simulink model "Model_14Bus_AC_DC_Microgrid"  (R2025a)
settings: Solver=ode23tb  StartTime=0.0  StopTime=0.1  MaxStep=1e-2  RelTol=1e-3
InitFcn:
  | Set_parameters_R2018
StopFcn:
  | Save_Data;
  | Graphics;
undefined symbols (not defined in the file): Clink, D1, Delta, dis1, dis10, dis11, dis12, dis13, dis14, dis2, dis3, dis4, dis5, dis6, dis7, dis8, dis9, Fc, Fnom, Hydride, Increment_MPPT, Ion, Ki_Ireg, Ki_VDCreg, Kp_Ireg, Kp_VDCreg, LimitL_Ireg, LimitL_VDCreg, Limits_MPPT, LimitU_Ireg, LimitU_VDCreg, Lithium, max_min, Metal, Nickel, P_Load_2, P_Load_3, Pnom, Pnom_T1, Pnom_T2, Pnom_T3, Pnom_xfo, Ql_Load_2, Ql_Load_3, R_Load_9, R_Load_DC, RL, Rl, RLff, Rls, sigbuilder_block, Ts, Ts_Control, Ts_Power, V1_LL_T3, Vf, Vfd, Vnom_dc, Vnom_DC, Vnom_Diesel ... (+5)
libraries: spsRMSLib x87, spsCurrentMeasurementLib x47, spsThreePhaseVIMeasurementLib x23, spsVoltageMeasurementLib x21, spsPowerLib x21, spsTHDLib x20, spsThreePhaseSeriesRLCBranchLib x20, spsSeriesRLCBranchLib x19, spsIGBTDiodeLib x14, spsThreePhaseBreakerLib x14, powerlib_extras x14, simulink x12
(part 4 of 9)

== system Model_14Bus_AC_DC_Microgrid/Bus_slack  ==
  note: C
  note: B
  note: A
  note: C
  note: Linea - Neutro
  note: B
  note: A
  note: A
  note: B
  note: C
  Conv pu1 : Gain  Gain=sqrt (3) /Vnom_prim  SaturateOnIntegerOverflow=on  OutDataTypeStr=Inherit: Same as input  ParamDataTypeStr=Inherit: Same as input
  Conv pu2 : Gain  Gain=sqrt (3) /Vnom_prim  SaturateOnIntegerOverflow=on  OutDataTypeStr=Inherit: Same as input  ParamDataTypeStr=Inherit: Same as input
  Measurement1 : Scope  NumInputPorts=4
      settings: SampleTime=Ts  Title=Active Powers (W)  ActiveDisplayYMinimum=-103868.59895  ActiveDisplayYMaximum=934817.39056  DataLoggingVariableName=ScopeData39  DataLoggingSaveFormat=Array
  PLL : Subsystem
  PLL (3ph) : spsPLL3phLib/PLL (3ph)  Fmin=45  Par_Init=[0, 60]  ParK=[180, 3200, 1]  TcD=1e-4  MaxRateChangeFreq=12  FilterCutOffFreq=25  Ts=0  AGC=on
  Power Factor Block1 : Subsystem  mask(Power Factor Block){Freq=Fnom, Vinit=[0, 0], Iinit=[0, 0], Ts=0}
      mask prompts: Freq "Fundamental frequency (Hz):"; Vinit "Voltage initial input [ Mag, Phase (degrees) ]:"; Iinit "Current initial input [ Mag, Phase (degrees) ]:"; Ts "Sample time:"
      mask help:
      | Power Factor Block developed by Dr Rodney Tan
      | Version 1.01 (Aug 2016)
      |
      | Compute power factor and phase angle of AC circuit voltage-current pair at fundamental frequency.
      |
      | The computation is based on Power block and Complex number function block.
      |
      | For the first cycle of simulation, the outputs are held constant to the powers computed for the Voltage initial input and Current initial input parameters.
      mask Help:
      | <b>Fundamental Frequency (Hz)</b>
      | Specify the measurement fundamental frequency, in hertz, of the input signal.
      | 
      | <b>Voltage initial input [ Mag, Phase (degrees) ]</b>
      | Specify the voltage initial magnitude and phase to set a constant output for the first cycle of simulation.
      | 
      | <b>Current initial input [ Mag, Phase (degrees) ]</b>
      | Specify the current initial magnitude and phase to set a constant output for the first cycle of simulation.
      | 
      | <b>Sample Time</b>
      | Specify the sample time of the block, in seconds. Set to 0 to implement a continuous block.
      mask TypeOptions Freq: Power/Freq
      mask TypeOptions Vinit: Power/Vinit
      mask TypeOptions Iinit: Power/Iinit
      mask TypeOptions Ts: Power/Ts
  Power Factor1 : Display
  Scope : Scope
      settings: ActiveDisplayYMinimum=-56.88569  ActiveDisplayYMaximum=237.8062
  Scope2 : Scope
      settings: DataLoggingVariableName=ScopeData3
  THD : spsTHDLib/THD  Freq=60  Ts=Ts_Power
  THD (% and signal) : Scope  NumInputPorts=2
      settings: TimeSpan=0.1  ActiveDisplayYMinimum=-21318.64578  ActiveDisplayYMaximum=21318.87173
  THD (%) : Display
      settings: Format=bank
  Terminator : Terminator
  Vabc pu1 : Scope
      settings: TimeSpan=3  Title=Vabc_Instantaneo y rms (pu)  ActiveDisplayYMinimum=-1.96658  ActiveDisplayYMaximum=2.46633  DataLoggingVariableName=ScopeData40
  frecuency (Hz) : Display
  to % : Gain  Gain=100  SampleTime=Ts_Power
  ángulo de V (%)1 : Display
      settings: Format=bank
  tag scope: PFabc_Bus13=global, THDv_abc_Bus13=global, delta_abc_Bus13=global
  wires:
  [Iabc_Sec] -> Power Factor Block1/2(Iabc)  "Signal Iabc"
  THD/1 -> to %/1
  Power Factor Block1/4(Iabc y Iabc (rms)) -> Measurement1/4
  Power Factor Block1/1(Pabc) -> Measurement1/1
  Conv pu1/1 -> Vabc pu1/1
  Power Factor Block1/2(Qabc) -> Measurement1/2
  Power Factor Block1/3(Vabc y Vabc (rms)) -> Conv pu1/1, Measurement1/3
  to %/1 -> [THDv_abc_Bus13], THD (%)/1, THD (% and signal)/2  "THD (%)"
  Power Factor Block1/5("PFabc ") -> [PFabc_Bus13], Power Factor1/1
  Conv pu2/1 -> PLL/1(Vabc_LN_pu)
  PLL/1(delta_abc) -> [delta_abc_Bus13], Scope/1, ángulo de V (%)1/1
  [Vabc_Sec] -> Power Factor Block1/1(Vabc), THD/1, THD (% and signal)/1, PLL (3ph)/1, Conv pu2/1  "Vabc"
  PLL (3ph)/2 -> Terminator/1
  PLL (3ph)/1 -> Scope2/1, frecuency (Hz)/1

== system Model_14Bus_AC_DC_Microgrid/Control measurement ==
  note: VL-L rms
  Bus Creator : BusCreator  Inputs=4
  VL-L : Scope  NumInputPorts=2
      settings: SampleTime=100e-6  TimeSpan=0.4  ActiveDisplayYMinimum=-206.95445  ActiveDisplayYMaximum=214.16347
  Vph_rms : Scope
      settings: SampleTime=100e-6  TimeSpan=0.4  ActiveDisplayYMinimum=-6.98302  ActiveDisplayYMaximum=62.8472
  m1 : Scope
      settings: SampleTime=100e-6  TimeSpan=0.04  ActiveDisplayYMinimum=-99.76377  ActiveDisplayYMaximum=99.5542
  measurement : Subsystem
  "                                          C" : PMIOPort  Side=Left
  "                                          B" : PMIOPort  Port=2  Side=Left
  "                                          A" : PMIOPort  Port=3  Side=Left
  "              Out1" : Outport  VectorParamsAs1DForOutWhenUnconnected=off
  wires:
  measurement/2(VL-L) -> VL-L/1, Bus Creator/2
  measurement/3(VL-L_rms) -> VL-L/2, Bus Creator/3
  measurement/4(Vph_rms) -> Vph_rms/1, Bus Creator/4
  measurement/1(Vph) -> m1/1, Bus Creator/1
  Bus Creator/1 -> "              Out1"/1
  connections:
  "                                          A"/RConn1 -- measurement/LConn1
  "                                          B"/RConn1 -- measurement/LConn2
  "                                          C"/RConn1 -- measurement/LConn3

== system Model_14Bus_AC_DC_Microgrid/Control measurement2 ==
  note: VL-L rms_3
  Bus Creator : BusCreator  Inputs=4
  VL-L_3 : Scope  NumInputPorts=2
      settings: SampleTime=100e-6  TimeSpan=0.4  ActiveDisplayYMinimum=-206.95445  ActiveDisplayYMaximum=214.16347  DataLoggingVariableName=ScopeData3
  Vph_rms_3 : Scope
      settings: SampleTime=100e-6  TimeSpan=0.4  ActiveDisplayYMinimum=-6.98302  ActiveDisplayYMaximum=62.8472  DataLoggingVariableName=ScopeData3
  m1_3 : Scope
      settings: SampleTime=100e-6  TimeSpan=0.04  ActiveDisplayYMinimum=-127.92327  ActiveDisplayYMaximum=126.27995  DataLoggingVariableName=ScopeData3
  measurement2 : Subsystem
  "                                          C" : PMIOPort  Side=Left
  "                                          B" : PMIOPort  Port=2  Side=Left
  "                                          A" : PMIOPort  Port=3  Side=Left
  "              Out1" : Outport  VectorParamsAs1DForOutWhenUnconnected=off
  wires:
  measurement2/2(VL-L) -> VL-L_3/1, Bus Creator/2
  measurement2/3(VL-L_rms) -> VL-L_3/2, Bus Creator/3
  measurement2/4(Vph_rms) -> Vph_rms_3/1, Bus Creator/4
  measurement2/1(Vph) -> m1_3/1, Bus Creator/1
  Bus Creator/1 -> "              Out1"/1
  connections:
  "                                          A"/RConn1 -- measurement2/LConn1
  "                                          B"/RConn1 -- measurement2/LConn2
  "                                          C"/RConn1 -- measurement2/LConn3

== system Model_14Bus_AC_DC_Microgrid/DATA  ADQUISITION ==
  note: Transformer (T1)
  note: Paper: "Hybrid AC/DC Microgrid test system simulation: Grid-connected mode"
  Delta_abc : Subsystem
  PF_abc : Subsystem
  P_abc : Subsystem
  Power_Losses_abc : Subsystem
  Q_abc : Subsystem
  RMS1 : spsRMSLib/RMS  TrueRMS=on  Freq=60  RMSInit=0  Ts=0
  RMS2 : spsRMSLib/RMS  TrueRMS=on  Freq=60  RMSInit=0  Ts=0
  THDv_abc : Subsystem
  VoltageLL_pu_abc : Subsystem
  scope 11 : Scope
      settings: TimeSpan=3  Title=Voltage  ActiveDisplayYMinimum=-0.12334  ActiveDisplayYMaximum=1.11006
  scope 12 : Scope
      settings: TimeSpan=3  Title=Voltage  ActiveDisplayYMinimum=-0.12406  ActiveDisplayYMaximum=1.11655  DataLoggingVariableName=ScopeData2
  wires:
  [Vabc_Sec_pu] -> RMS1/1
  RMS1/1 -> scope 11/1
  RMS2/1 -> scope 12/1
  [Vabc_Prim_pu] -> RMS2/1  "Signal Vabc"

== system Model_14Bus_AC_DC_Microgrid/Diesel_ 3MVA ==
  note: Diesel generator 2
  2.4kV  50MVA : spsThreePhaseSeriesRLCBranchLib/Three-Phase Series RLC Branch  LConnTagsString=A|B|C  RConnTagsString=A|B|C  BranchType=RL  Resistance=2.4e3^2/50e6/10  Inductance=2.4e3^2/50e6/(2*pi*60)  Capacitance=1.0  Measurements=None
  Ground1 : spsGroundLib/Ground  LConnTagsString=a
  Programmable Voltage Source1 : spsThreePhaseProgrammableVoltageSourceLib/Three-Phase Programmable Voltage Source  PositiveSequence="[Vnom_Diesel*0.9848 -60  Fnom]"  VariationEntity=None  VariationType=Table of time-amplitude pairs  VariationTypeAlt=Step  VariationStep=-0.3  VariationRate=0.5  VariationMagnitude=0.4  VariationFrequency=2  VariationTiming=[0.1 1.2]  VariationPhaseA=off  Amplitudes=[1]  TimeValues=[0]  HarmonicGeneration=off  HarmonicA=[3 0.2 -25 0]  HarmonicB="[2 0.15  35 2]"  Timing="[0.1  0.6]"  BusType=PV  Pref=Pgen_Diesel  Qref=0  Qmin=-inf  Qmax=inf
  a1 : PMIOPort  Tag=PMCPort  Side=Left
  b1 : PMIOPort  Tag=PMCPort  Port=2  Side=Left
  c1 : PMIOPort  Tag=PMCPort  Port=3  Side=Left
  connections:
  Programmable Voltage Source1/RConn3 -- 2.4kV  50MVA/LConn3
  Ground1/LConn1 -- Programmable Voltage Source1/LConn1
  Programmable Voltage Source1/RConn2 -- 2.4kV  50MVA/LConn2
  2.4kV  50MVA/LConn1 -- Programmable Voltage Source1/RConn1
  b1/RConn1 -- 2.4kV  50MVA/RConn2
  a1/RConn1 -- 2.4kV  50MVA/RConn1
  c1/RConn1 -- 2.4kV  50MVA/RConn3

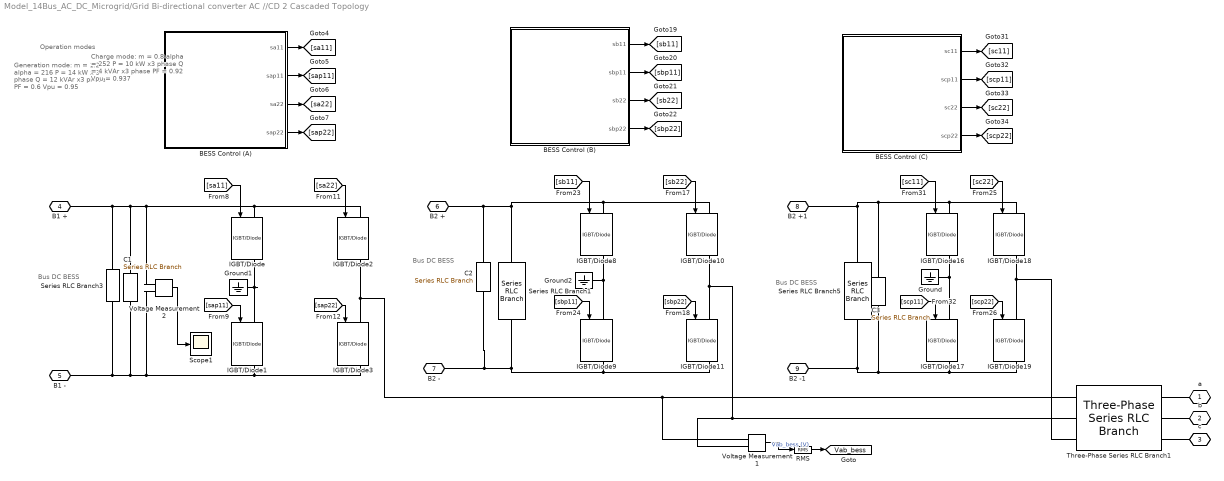
== system Model_14Bus_AC_DC_Microgrid/Grid Bi-directional converter AC //CD 2 Cascaded Topology ==
  note: Operation modes
  note: Generation mode:
      |
      | m = 1.2
      | alpha = 216
      |
      | P = 14 kW x 3 phase
      | Q = 12 kVAr x3 phase
      | PF = 0.6
      | Vpu = 0.95
  note: Bus DC BESS
  note: Bus DC BESS
  note: Bus DC BESS
  note: Charge mode:
      |
      | m = 0.8
      | alpha = 252
      |
      | P = 10 kW x3 phase
      | Q = 4 kVAr x3 phase
      | PF = 0.92
      | Vpu = 0.937
  BESS Control (A) : Subsystem
      mask Display: image('Icons\FPGA.png');
  BESS Control (B) : Subsystem
      mask Display: image('Icons\FPGA.png');
  BESS Control (C) : Subsystem
      mask Display: image('Icons\FPGA.png');
  C1 : spsSeriesRLCBranchLib/Series RLC Branch  LConnTagsString=__new0  RConnTagsString=__new0  BranchType=C  Resistance=22.5  Inductance=1e-3  SetiL0=off  InitialCurrent=0  Capacitance=10e-3  Setx0=off  InitialVoltage=0  Measurements=None
  C2 : spsSeriesRLCBranchLib/Series RLC Branch  LConnTagsString=__new0  RConnTagsString=__new0  BranchType=C  Resistance=22.5  Inductance=1e-3  SetiL0=off  InitialCurrent=0  Capacitance=10e-3  Setx0=off  InitialVoltage=0  Measurements=None
  C3 : spsSeriesRLCBranchLib/Series RLC Branch  LConnTagsString=__new0  RConnTagsString=__new0  BranchType=C  Resistance=22.5  Inductance=1e-3  SetiL0=off  InitialCurrent=0  Capacitance=10e-3  Setx0=off  InitialVoltage=0  Measurements=None
  Ground : spsGroundLib/Ground  LConnTagsString=a
  Ground1 : spsGroundLib/Ground  LConnTagsString=a
  Ground2 : spsGroundLib/Ground  LConnTagsString=a
  IGBT/Diode{,1..3,8..11,16..19} (12 alike) : spsIGBTDiodeLib/IGBT//Diode  Ron=1e-3  Rs=1e5  Cs=inf  Measurements=on
  RMS : spsRMSLib/RMS  TrueRMS=off  Freq=60  RMSInit=1  Ts=0
  Scope1 : Scope
      settings: ActiveDisplayYMinimum=-148.30159  ActiveDisplayYMaximum=1335.16158
  Series RLC Branch1 : spsSeriesRLCBranchLib/Series RLC Branch  LConnTagsString=__new0  RConnTagsString=__new0  BranchType=R  Resistance=1e9  Inductance=1e-3  SetiL0=off  InitialCurrent=0  Capacitance=1e-6  Setx0=off  InitialVoltage=0  Measurements=None
  Series RLC Branch3 : spsSeriesRLCBranchLib/Series RLC Branch  LConnTagsString=__new0  RConnTagsString=__new0  BranchType=R  Resistance=1e9  Inductance=1e-3  SetiL0=off  InitialCurrent=0  Capacitance=1e-6  Setx0=off  InitialVoltage=0  Measurements=None
  Series RLC Branch5 : spsSeriesRLCBranchLib/Series RLC Branch  LConnTagsString=__new0  RConnTagsString=__new0  BranchType=R  Resistance=1e9  Inductance=1e-3  SetiL0=off  InitialCurrent=0  Capacitance=1e-6  Setx0=off  InitialVoltage=0  Measurements=None
  Three-Phase Series RLC Branch1 : spsThreePhaseSeriesRLCBranchLib/Three-Phase Series RLC Branch  LConnTagsString=A|B|C  RConnTagsString=A|B|C  BranchType=RL  Resistance=1  Inductance=1.2e-2  Capacitance=15.5e-5  Measurements=None
  Voltage Measurement1 : spsVoltageMeasurementLib/Voltage Measurement  PhasorSimulation=off  OutputType=Complex  PSBequivalent=0
  Voltage Measurement2 : spsVoltageMeasurementLib/Voltage Measurement  PhasorSimulation=off  OutputType=Complex  PSBequivalent=0
  "a " : PMIOPort  Tag=PMCPort  Side=Left
  b : PMIOPort  Tag=PMCPort  Port=2  Side=Left
  c : PMIOPort  Tag=PMCPort  Port=3  Side=Left
  B1 + : PMIOPort  Port=4  Side=Right
  B1 - : PMIOPort  Port=5  Side=Right
  B2 + : PMIOPort  Port=6  Side=Right
  B2 - : PMIOPort  Port=7  Side=Right
  B2 +1 : PMIOPort  Port=8  Side=Right
  B2 -1 : PMIOPort  Port=9  Side=Right
  tag scope: Vab_bess=global
  wires:
  [sa11] -> IGBT/Diode/1
  [sap11] -> IGBT/Diode1/1
  [sa22] -> IGBT/Diode2/1
  [sap22] -> IGBT/Diode3/1
  [sb11] -> IGBT/Diode8/1
  [sbp11] -> IGBT/Diode9/1
  [sb22] -> IGBT/Diode10/1
  [sbp22] -> IGBT/Diode11/1
  [sc11] -> IGBT/Diode16/1
  [scp11] -> IGBT/Diode17/1
  [sc22] -> IGBT/Diode18/1
  [scp22] -> IGBT/Diode19/1
  Voltage Measurement1/1 -> RMS/1  "Vab_bess (V)"
  RMS/1 -> [Vab_bess]
  Voltage Measurement2/1 -> Scope1/1
  BESS Control (A)/1(sa11) -> [sa11]
  BESS Control (A)/2(sap11) -> [sap11]
  BESS Control (A)/3(sa22) -> [sa22]
  BESS Control (A)/4(sap22) -> [sap22]
  BESS Control (B)/1(sb11) -> [sb11]
  BESS Control (B)/2(sbp11) -> [sbp11]
  BESS Control (B)/3(sb22) -> [sb22]
  BESS Control (B)/4(sbp22) -> [sbp22]
  BESS Control (C)/1(sc11) -> [sc11]
  BESS Control (C)/2(scp11) -> [scp11]
  BESS Control (C)/3(sc22) -> [sc22]
  BESS Control (C)/4(scp22) -> [scp22]
  connections:
  IGBT/Diode1/RConn1 -- IGBT/Diode3/RConn1 -- C1/RConn1 -- Series RLC Branch3/RConn1 -- B1 -/RConn1 -- Voltage Measurement2/LConn2
  Series RLC Branch1/RConn1 -- C2/RConn1 -- B2 -/RConn1 -- IGBT/Diode9/RConn1 -- IGBT/Diode11/RConn1
  IGBT/Diode11/LConn1 -- Voltage Measurement1/LConn2 -- Three-Phase Series RLC Branch1/LConn2 -- IGBT/Diode10/RConn1
  Series RLC Branch5/RConn1 -- B2 -1/RConn1 -- C3/RConn1 -- IGBT/Diode19/RConn1 -- IGBT/Diode17/RConn1
  IGBT/Diode19/LConn1 -- Three-Phase Series RLC Branch1/LConn3 -- IGBT/Diode18/RConn1
  IGBT/Diode/LConn1 -- IGBT/Diode2/LConn1 -- Voltage Measurement2/LConn1 -- C1/LConn1 -- B1 +/RConn1 -- Series RLC Branch3/LConn1
  Voltage Measurement1/LConn1 -- IGBT/Diode2/RConn1 -- IGBT/Diode3/LConn1 -- Three-Phase Series RLC Branch1/LConn1
  IGBT/Diode8/LConn1 -- C2/LConn1 -- B2 +/RConn1 -- Series RLC Branch1/LConn1 -- IGBT/Diode10/LConn1
  IGBT/Diode16/LConn1 -- C3/LConn1 -- Series RLC Branch5/LConn1 -- B2 +1/RConn1 -- IGBT/Diode18/LConn1
  IGBT/Diode1/LConn1 -- Ground1/LConn1 -- IGBT/Diode/RConn1
  IGBT/Diode9/LConn1 -- Ground2/LConn1 -- IGBT/Diode8/RConn1
  IGBT/Diode16/RConn1 -- Ground/LConn1 -- IGBT/Diode17/LConn1
  "a "/RConn1 -- Three-Phase Series RLC Branch1/RConn1
  b/RConn1 -- Three-Phase Series RLC Branch1/RConn2
  c/RConn1 -- Three-Phase Series RLC Branch1/RConn3

== system Model_14Bus_AC_DC_Microgrid/Grid Bi-directional Converter 1.1 300 (DC) // 150 V (AC) P_nom 3kW ==
  note: Bus DC
  note: Bus AC
  note: Inverter mode:
      |
      | m = 1.2
      | alpha = 0
      |
      | P = 1 kW x 3 phase
      | Q = 1 kVAr x3 phase
      | PF = 0.6
      | Vpu = 0.95
  note: Operation modes
  note: Rectif mode:
      |
      | m = 1
      | alpha = 228
      |
      | P = 975 kVA (DC)
  Means : Inport
  C1 : spsSeriesRLCBranchLib/Series RLC Branch  LConnTagsString=__new0  RConnTagsString=__new0  BranchType=C  Resistance=22.5  Inductance=1e-3  SetiL0=off  InitialCurrent=0  Capacitance=1200e-6  Setx0=off  InitialVoltage=150  Measurements=None
  Control of Inverter : Subsystem
      mask Display: image('Icons\FPGA.png');
  Ground1 : spsGroundLib/Ground  LConnTagsString=a
  Scope : Scope
      settings: ActiveDisplayYMinimum=-0.125  ActiveDisplayYMaximum=1.125  DataLoggingVariableName=ScopeData2
  Three-Phase Parallel RLC Branch1 : spsThreePhaseParallelRLCBranchLib/Three-Phase Parallel RLC Branch  LConnTagsString=A|B|C  RConnTagsString=A|B|C  BranchType=C  Resistance=1  Inductance=1e-3  Capacitance=2.65e-6  Measurements=None
  Three-Phase Series RLC Branch1 : spsThreePhaseSeriesRLCBranchLib/Three-Phase Series RLC Branch  LConnTagsString=A|B|C  RConnTagsString=A|B|C  BranchType=RL  Resistance=2  Inductance=1e-2  Capacitance=15.5e-5  Measurements=None
  Universal Bridge1 : spsUniversalBridgeLib/Universal Bridge  Arms=3  SnubberResistance=1e5  SnubberCapacitance=inf  Device=MOSFET / Diodes  Ron=1e-3  Lon=0  ForwardVoltages="[  0  0  ]"  ForwardVoltage=0  GTOparameters=[ 10e-6 , 20e-6 ]  IGBTparameters=[ 1e-6 , 2e-6 ]  Measurements=None  Measurements_2=None  converterType=Rectifier
  "a " : PMIOPort  Tag=PMCPort  Side=Left
  b : PMIOPort  Tag=PMCPort  Port=2  Side=Left
  c : PMIOPort  Tag=PMCPort  Port=3  Side=Left
  B1 + : PMIOPort  Port=4  Side=Right
  B1 - : PMIOPort  Port=5  Side=Right
  tag scope: Pulse=global
  wires:
  Control of Inverter/1(Pulses) -> Scope/1, [Pulse]
  [Pulse] -> Universal Bridge1/1
  Means/1 -> Control of Inverter/1(Means)
  connections:
  Three-Phase Series RLC Branch1/RConn1 -- Three-Phase Parallel RLC Branch1/LConn1 -- "a "/RConn1
  Three-Phase Parallel RLC Branch1/LConn2 -- Three-Phase Series RLC Branch1/RConn2 -- b/RConn1
  Three-Phase Parallel RLC Branch1/LConn3 -- Three-Phase Series RLC Branch1/RConn3 -- c/RConn1
  Ground1/LConn1 -- Three-Phase Parallel RLC Branch1/RConn3 -- Three-Phase Parallel RLC Branch1/RConn1 -- Three-Phase Parallel RLC Branch1/RConn2
  Universal Bridge1/LConn3 -- Three-Phase Series RLC Branch1/LConn3
  Three-Phase Series RLC Branch1/LConn2 -- Universal Bridge1/LConn2
  Universal Bridge1/LConn1 -- Three-Phase Series RLC Branch1/LConn1
  B1 +/RConn1 -- C1/LConn1 -- Universal Bridge1/RConn1
  B1 -/RConn1 -- C1/RConn1 -- Universal Bridge1/RConn2

== system Model_14Bus_AC_DC_Microgrid/Grid Bi-directional Converter 1.2 300 (DC) // 150 V (AC) P_nom 3kW ==
  note: DC Bus
  note: AC Bus
  note: Inverter mode:
      |
      | m = 1.2
      | alpha = 0
      |
      | P = 1 kW x 3 phase
      | Q = 1 kVAr x3 phase
      | PF = 0.6
      | Vpu = 0.95
  note: Rectif mode:
      |
      | NO WORK
  Means2 : Inport
  C1 : spsSeriesRLCBranchLib/Series RLC Branch  LConnTagsString=__new0  RConnTagsString=__new0  BranchType=C  Resistance=22.5  Inductance=1e-3  SetiL0=off  InitialCurrent=0  Capacitance=1200e-6  Setx0=off  InitialVoltage=150  Measurements=None
  Control of Inverter : Subsystem
      mask Display: image('Icons\FPGA.png');
  Ground1 : spsGroundLib/Ground  LConnTagsString=a
  Scope : Scope
      settings: ActiveDisplayYMinimum=-0.125  ActiveDisplayYMaximum=1.125
  Three-Phase Parallel RLC Branch2 : spsThreePhaseParallelRLCBranchLib/Three-Phase Parallel RLC Branch  LConnTagsString=A|B|C  RConnTagsString=A|B|C  BranchType=C  Resistance=1  Inductance=1e-3  Capacitance=2.65e-6  Measurements=None
  Three-Phase Series RLC Branch2 : spsThreePhaseSeriesRLCBranchLib/Three-Phase Series RLC Branch  LConnTagsString=A|B|C  RConnTagsString=A|B|C  BranchType=RL  Resistance=2  Inductance=1e-2  Capacitance=15.5e-5  Measurements=None
  Universal Bridge2 : spsUniversalBridgeLib/Universal Bridge  Arms=3  SnubberResistance=1e5  SnubberCapacitance=inf  Device=MOSFET / Diodes  Ron=1e-3  Lon=0  ForwardVoltages="[  0  0  ]"  ForwardVoltage=0  GTOparameters=[ 10e-6 , 20e-6 ]  IGBTparameters=[ 1e-6 , 2e-6 ]  Measurements=None  Measurements_2=None  converterType=Rectifier
  "a " : PMIOPort  Tag=PMCPort  Side=Left
  b : PMIOPort  Tag=PMCPort  Port=2  Side=Left
  c : PMIOPort  Tag=PMCPort  Port=3  Side=Left
  B1 + : PMIOPort  Port=4  Side=Right
  B1 - : PMIOPort  Port=5  Side=Right
  tag scope: Pulse2=global
  wires:
  Control of Inverter/1(Pulses) -> Scope/1, [Pulse2]
  Means2/1 -> Control of Inverter/1(Means2)
  [Pulse2] -> Universal Bridge2/1
  connections:
  Three-Phase Series RLC Branch2/RConn1 -- Three-Phase Parallel RLC Branch2/LConn1 -- "a "/RConn1
  Three-Phase Parallel RLC Branch2/LConn2 -- Three-Phase Series RLC Branch2/RConn2 -- b/RConn1
  Three-Phase Parallel RLC Branch2/LConn3 -- Three-Phase Series RLC Branch2/RConn3 -- c/RConn1
  Ground1/LConn1 -- Three-Phase Parallel RLC Branch2/RConn3 -- Three-Phase Parallel RLC Branch2/RConn1 -- Three-Phase Parallel RLC Branch2/RConn2
  Universal Bridge2/LConn3 -- Three-Phase Series RLC Branch2/LConn3
  Three-Phase Series RLC Branch2/LConn2 -- Universal Bridge2/LConn2
  Universal Bridge2/LConn1 -- Three-Phase Series RLC Branch2/LConn1
  Universal Bridge2/RConn1 -- B1 +/RConn1 -- C1/LConn1
  B1 -/RConn1 -- Universal Bridge2/RConn2 -- C1/RConn1

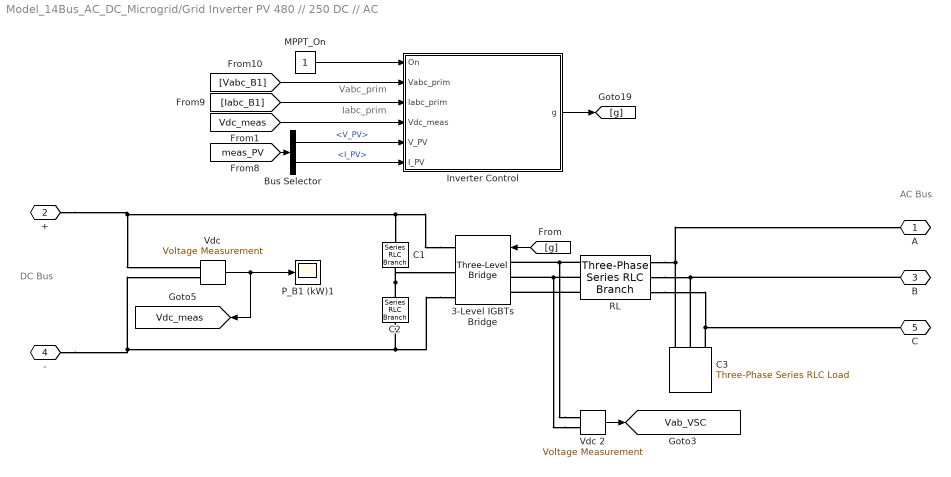
== system Model_14Bus_AC_DC_Microgrid/Grid Inverter PV 480 // 250 DC // AC  ==
  note: Iabc_prim
  note: Vabc_prim
  note: AC Bus
  note: DC Bus
  3-Level IGBTs Bridge : spsThreeLevelBridgeLib/Three-Level Bridge  Arms=3  SnubberResistance=Rs  SbubberCapacitance=Cs  Device=IGBT / Diodes  Ron=Ron  ForwardVoltages="[  Vfd  Vf ]"  Measurements=None
      settings: AttributesFormatString=\n  LibrarySourceBlock=sps_lib/Power Electronics/Three-Level Bridge
  Bus Selector : BusSelector  OutputSignals=V_PV,I_PV
  C1 : spsSeriesRLCBranchLib/Series RLC Branch  LConnTagsString=__new0  RConnTagsString=__new0  BranchType=C  Resistance=1.0  Inductance=1.0  SetiL0=off  InitialCurrent=0  Capacitance=Clink  Setx0=on  InitialVoltage=Vnom_dc/2  Measurements=None
  C2 : spsSeriesRLCBranchLib/Series RLC Branch  LConnTagsString=__new0  RConnTagsString=__new0  BranchType=C  Resistance=1.0  Inductance=1.0  SetiL0=off  InitialCurrent=0  Capacitance=Clink  Setx0=on  InitialVoltage=Vnom_dc/2  Measurements=None
  C3 : spsThreePhaseSeriesRLCLoadLib/Three-Phase Series RLC Load  LConnTagsString=A|B|C  Configuration=Delta  NominalVoltage=Vnom_sec  Vabc=[1e3 1e3 1e3]  Vabcp=[1e3 1e3 1e3]  NominalFrequency=Fnom  UnbalancedPower=off  ActivePower=Pc  InductivePower=0  CapacitivePower=Qc  Pabc=[10e3 9e3 11e3]  QLabc=[100 90 110]  QCabc=[100 90 110]  Pabcp=[10e3 9e3 11e3]  QLabcp=[100 90 110]  QCabcp=[100 90 110]  Measurements=None  LoadType=constant Z
  Inverter Control : Subsystem  mask(Inverter Control){Pnom=Pnom, Fnom=Fnom, Vnom_prim=Vnom_prim, Vnom_sec=Vnom_sec, Vnom_dc=Vnom_dc, Increment_MPPT=Increment_MPPT, Limits_MPPT=Limits_MPPT, Vdc_ref_Init=Vnom_dc, Kp_VDCreg=Kp_VDCreg, Ki_VDCreg=Ki_VDCreg, Kp_Ireg=Kp_Ireg, Ki_Ireg=Ki_Ireg, RLff=RLff, Fc=Fc, Ts_Control=Ts_Control, Ts_PWMgenerator=Ts_Power}
      mask prompts: Pnom "Power (VA)"; Fnom "Frequency (Hz)"; Vnom_prim "Primary voltage (Vrms LL)"; Vnom_sec "Secondary voltage (Vrms LL)"; Vnom_dc "DC voltage (V)"; Increment_MPPT "Output increment (V)"; Limits_MPPT "Output limits [ Upper  Lower ]"; Vdc_ref_Init "Output initial value (V)"; Kp_VDCreg "Proportional gain"; Ki_VDCreg "Integral gain"; Kp_Ireg "Proportional gain"; Ki_Ireg "Integral gain"; RLff "Feedforward Values [Rff Lff]"; Fc "Carrier frequency (Hz)"; Ts_Control "Control systems"; Ts_PWMgenerator "PWM generator"
      mask help:
      | The main components of the Inverter Control are:
      | 1. PLL & Measurements
      | 2. Maximum Power Point Tracker System (MPPT) using a Perturb & Observe algorithm
      | 3. DC Voltage Regulator
      | 4. Current Regulator
      | 5. PWM Modulator
      mask DialogControl Container4 Prompt: Nominal Values:
      mask DialogControl Container3 Prompt: MPPT Controller:
      mask DialogControl Container8 Prompt: Dc Voltage Regulator:
      mask DialogControl Container6 Prompt: Current Regulator:
      mask DialogControl Container9 Prompt: PWM Modulator:
      mask DialogControl SampleTimes Prompt: Sample Times:
      mask Display: image('Icons\FPGA.png');
  MPPT_On : Constant
  P_B1 (kW)1 : Scope
      settings: ActiveDisplayYMinimum=454.62824  ActiveDisplayYMaximum=525.40165  DataLoggingVariableName=ScopeData6
  RL : spsThreePhaseSeriesRLCBranchLib/Three-Phase Series RLC Branch  LConnTagsString=A|B|C  RConnTagsString=A|B|C  BranchType=RL  Resistance=RL(1)  Inductance=RL(2)  Capacitance=inf  Measurements=None
  "Vdc " : spsVoltageMeasurementLib/Voltage Measurement  Tag=PoWeRsYsTeMmEaSuReMeNt  PhasorSimulation=off  OutputType=Magnitude  PSBequivalent=0
  Vdc 2 : spsVoltageMeasurementLib/Voltage Measurement  Tag=PoWeRsYsTeMmEaSuReMeNt  PhasorSimulation=off  OutputType=Magnitude  PSBequivalent=0
  A : PMIOPort  Side=Right
  + : PMIOPort  Port=2  Side=Left
  B : PMIOPort  Port=3  Side=Right
  - : PMIOPort  Port=4  Side=Left
  C : PMIOPort  Port=5  Side=Right
  tag scope: Vab_VSC=global, Vdc_meas=global
  wires:
  Bus Selector/1 -> Inverter Control/5(V_PV)  "<V_PV>"
  [Vdc_meas] -> Inverter Control/4(Vdc_meas)
  [meas_PV] -> Bus Selector/1
  MPPT_On/1 -> Inverter Control/1(On)
  [Vabc_B1] -> Inverter Control/2(Vabc_prim)
  [Iabc_B1] -> Inverter Control/3(Iabc_prim)
  Bus Selector/2 -> Inverter Control/6(I_PV)  "<I_PV>"
  "Vdc "/1 -> [Vdc_meas], P_B1 (kW)1/1
  Vdc 2/1 -> [Vab_VSC]
  Inverter Control/1(g) -> [g]
  [g] -> 3-Level IGBTs Bridge/1
  connections:
  Vdc 2/LConn1 -- 3-Level IGBTs Bridge/LConn1 -- RL/LConn1
  Vdc 2/LConn2 -- 3-Level IGBTs Bridge/LConn2 -- RL/LConn2
  C3/LConn1 -- RL/RConn1 -- A/RConn1
  C3/LConn2 -- RL/RConn2 -- B/RConn1
  3-Level IGBTs Bridge/RConn3 -- -/RConn1 -- "Vdc "/LConn2 -- C2/RConn1
  C1/RConn1 -- C2/LConn1 -- 3-Level IGBTs Bridge/RConn2
  3-Level IGBTs Bridge/RConn1 -- C1/LConn1 -- "Vdc "/LConn1 -- +/RConn1
  RL/LConn3 -- 3-Level IGBTs Bridge/LConn3
  C3/LConn3 -- RL/RConn3 -- C/RConn1

== system Model_14Bus_AC_DC_Microgrid/Load_1 ==
  note: C
  note: Linea - Neutro
  note: B
  note: A
  Conv pu1 : Gain  Gain=sqrt (3) /Vnom_sec  SaturateOnIntegerOverflow=on  OutDataTypeStr=Inherit: Same as input  ParamDataTypeStr=Inherit: Same as input
  Measurement1 : Scope  NumInputPorts=4
      settings: SampleTime=Ts  Title=Active Powers (W)  ActiveDisplayYMinimum=-5269.67563  ActiveDisplayYMaximum=47427.08071  DataLoggingVariableName=ScopeData21  DataLoggingSaveFormat=Array
  Power Factor Block1 : Subsystem  mask(Power Factor Block){Freq=Fnom, Vinit=[0, 0], Iinit=[0, 0], Ts=0}
      mask prompts: Freq "Fundamental frequency (Hz):"; Vinit "Voltage initial input [ Mag, Phase (degrees) ]:"; Iinit "Current initial input [ Mag, Phase (degrees) ]:"; Ts "Sample time:"
      mask help:
      | Power Factor Block developed by Dr Rodney Tan
      | Version 1.01 (Aug 2016)
      |
      | Compute power factor and phase angle of AC circuit voltage-current pair at fundamental frequency.
      |
      | The computation is based on Power block and Complex number function block.
      |
      | For the first cycle of simulation, the outputs are held constant to the powers computed for the Voltage initial input and Current initial input parameters.
      mask Help:
      | <b>Fundamental Frequency (Hz)</b>
      | Specify the measurement fundamental frequency, in hertz, of the input signal.
      | 
      | <b>Voltage initial input [ Mag, Phase (degrees) ]</b>
      | Specify the voltage initial magnitude and phase to set a constant output for the first cycle of simulation.
      | 
      | <b>Current initial input [ Mag, Phase (degrees) ]</b>
      | Specify the current initial magnitude and phase to set a constant output for the first cycle of simulation.
      | 
      | <b>Sample Time</b>
      | Specify the sample time of the block, in seconds. Set to 0 to implement a continuous block.
      mask TypeOptions Freq: Power/Freq
      mask TypeOptions Vinit: Power/Vinit
      mask TypeOptions Iinit: Power/Iinit
      mask TypeOptions Ts: Power/Ts
  Power Factor1 : Display
  Vabc pu1 : Scope
      settings: TimeSpan=3  Title=Vabc_Instantaneo y rms (pu)  ActiveDisplayYMinimum=-1.71551  ActiveDisplayYMaximum=1.71557  DataLoggingVariableName=ScopeData22
  wires:
  [Iabc_load_1] -> Power Factor Block1/2(Iabc)
  [Vabc_load_1] -> Power Factor Block1/1(Vabc)
  Power Factor Block1/4(Iabc y Iabc (rms)) -> Measurement1/4
  Power Factor Block1/1(Pabc) -> Measurement1/1
  Conv pu1/1 -> Vabc pu1/1
  Power Factor Block1/5("PFabc ") -> Power Factor1/1
  Power Factor Block1/2(Qabc) -> Measurement1/2
  Power Factor Block1/3(Vabc y Vabc (rms)) -> Conv pu1/1, Measurement1/3

== system Model_14Bus_AC_DC_Microgrid/Load_2 ==
  note: C
  note: B
  note: A
  note: C
  note: Linea - Neutro
  note: B
  note: A
  Conv pu1 : Gain  Gain=sqrt (3) /Vnom_sec  SaturateOnIntegerOverflow=on  OutDataTypeStr=Inherit: Same as input  ParamDataTypeStr=Inherit: Same as input
  Measurement1 : Scope  NumInputPorts=4
      settings: SampleTime=Ts  Title=Active Powers (W)  ActiveDisplayYMinimum=-2870.82629  ActiveDisplayYMaximum=25837.43663  DataLoggingVariableName=ScopeData17  DataLoggingSaveFormat=Array
  Power Factor Block1 : Subsystem  mask(Power Factor Block){Freq=Fnom, Vinit=[0, 0], Iinit=[0, 0], Ts=0}
      mask prompts: Freq "Fundamental frequency (Hz):"; Vinit "Voltage initial input [ Mag, Phase (degrees) ]:"; Iinit "Current initial input [ Mag, Phase (degrees) ]:"; Ts "Sample time:"
      mask help:
      | Power Factor Block developed by Dr Rodney Tan
      | Version 1.01 (Aug 2016)
      |
      | Compute power factor and phase angle of AC circuit voltage-current pair at fundamental frequency.
      |
      | The computation is based on Power block and Complex number function block.
      |
      | For the first cycle of simulation, the outputs are held constant to the powers computed for the Voltage initial input and Current initial input parameters.
      mask Help:
      | <b>Fundamental Frequency (Hz)</b>
      | Specify the measurement fundamental frequency, in hertz, of the input signal.
      | 
      | <b>Voltage initial input [ Mag, Phase (degrees) ]</b>
      | Specify the voltage initial magnitude and phase to set a constant output for the first cycle of simulation.
      | 
      | <b>Current initial input [ Mag, Phase (degrees) ]</b>
      | Specify the current initial magnitude and phase to set a constant output for the first cycle of simulation.
      | 
      | <b>Sample Time</b>
      | Specify the sample time of the block, in seconds. Set to 0 to implement a continuous block.
      mask TypeOptions Freq: Power/Freq
      mask TypeOptions Vinit: Power/Vinit
      mask TypeOptions Iinit: Power/Iinit
      mask TypeOptions Ts: Power/Ts
  Power Factor1 : Display
  THD : spsTHDLib/THD  Freq=60  Ts=Ts_Power
  THD (% and signal) : Scope  NumInputPorts=2
      settings: TimeSpan=0.1  ActiveDisplayYMinimum=-236.74679  ActiveDisplayYMaximum=236.7544  DataLoggingVariableName=ScopeData13
  THD (%) : Display
      settings: Format=bank
  Vabc pu1 : Scope
      settings: TimeSpan=3  Title=Vabc_Instantaneo y rms (pu)  ActiveDisplayYMinimum=-1.70857  ActiveDisplayYMaximum=1.70863  DataLoggingVariableName=ScopeData18
  to % : Gain  Gain=100  SampleTime=Ts_Power
  wires:
  [Iabc_load_2] -> Power Factor Block1/2(Iabc)
  [Vabc_load_2] -> Power Factor Block1/1(Vabc), THD/1, THD (% and signal)/1  "Signal Vabc"
  THD/1 -> to %/1
  to %/1 -> THD (%)/1, THD (% and signal)/2  "THD (%)"
  Power Factor Block1/4(Iabc y Iabc (rms)) -> Measurement1/4
  Power Factor Block1/1(Pabc) -> Measurement1/1
  Conv pu1/1 -> Vabc pu1/1
  Power Factor Block1/5("PFabc ") -> Power Factor1/1
  Power Factor Block1/2(Qabc) -> Measurement1/2
  Power Factor Block1/3(Vabc y Vabc (rms)) -> Conv pu1/1, Measurement1/3

== system Model_14Bus_AC_DC_Microgrid/Load_3 ==
  note: C
  note: B
  note: A
  note: C
  note: Linea - Neutro
  note: B
  note: A
  Conv pu1 : Gain  Gain=sqrt (3) /Vnom_prim  SaturateOnIntegerOverflow=on  OutDataTypeStr=Inherit: Same as input  ParamDataTypeStr=Inherit: Same as input
  Measurement1 : Scope  NumInputPorts=4
      settings: SampleTime=Ts  Title=Active Powers (W)  ActiveDisplayYMinimum=-15812.29037  ActiveDisplayYMaximum=142310.61332  DataLoggingVariableName=ScopeData17  DataLoggingSaveFormat=Array
  Power Factor Block1 : Subsystem  mask(Power Factor Block){Freq=Fnom, Vinit=[0, 0], Iinit=[0, 0], Ts=0}
      mask prompts: Freq "Fundamental frequency (Hz):"; Vinit "Voltage initial input [ Mag, Phase (degrees) ]:"; Iinit "Current initial input [ Mag, Phase (degrees) ]:"; Ts "Sample time:"
      mask help:
      | Power Factor Block developed by Dr Rodney Tan
      | Version 1.01 (Aug 2016)
      |
      | Compute power factor and phase angle of AC circuit voltage-current pair at fundamental frequency.
      |
      | The computation is based on Power block and Complex number function block.
      |
      | For the first cycle of simulation, the outputs are held constant to the powers computed for the Voltage initial input and Current initial input parameters.
      mask Help:
      | <b>Fundamental Frequency (Hz)</b>
      | Specify the measurement fundamental frequency, in hertz, of the input signal.
      | 
      | <b>Voltage initial input [ Mag, Phase (degrees) ]</b>
      | Specify the voltage initial magnitude and phase to set a constant output for the first cycle of simulation.
      | 
      | <b>Current initial input [ Mag, Phase (degrees) ]</b>
      | Specify the current initial magnitude and phase to set a constant output for the first cycle of simulation.
      | 
      | <b>Sample Time</b>
      | Specify the sample time of the block, in seconds. Set to 0 to implement a continuous block.
      mask TypeOptions Freq: Power/Freq
      mask TypeOptions Vinit: Power/Vinit
      mask TypeOptions Iinit: Power/Iinit
      mask TypeOptions Ts: Power/Ts
  Power Factor1 : Display
  THD : spsTHDLib/THD  Freq=60  Ts=Ts_Power
  THD (% and signal) : Scope  NumInputPorts=2
      settings: TimeSpan=0.1  ActiveDisplayYMinimum=-236.74679  ActiveDisplayYMaximum=236.7544  DataLoggingVariableName=ScopeData13
  THD (%) : Display
      settings: Format=bank
  Vabc pu1 : Scope
      settings: TimeSpan=3  Title=Vabc_Instantaneo y rms (pu)  ActiveDisplayYMinimum=-2.08414  ActiveDisplayYMaximum=2.62408  DataLoggingVariableName=ScopeData18
  to % : Gain  Gain=100  SampleTime=Ts_Power
  wires:
  [Iabc_load_14] -> Power Factor Block1/2(Iabc)
  [Vabc_load_14] -> Power Factor Block1/1(Vabc), THD/1, THD (% and signal)/1  "Signal Vabc"
  THD/1 -> to %/1
  to %/1 -> THD (%)/1, THD (% and signal)/2  "THD (%)"
  Power Factor Block1/4(Iabc y Iabc (rms)) -> Measurement1/4
  Power Factor Block1/1(Pabc) -> Measurement1/1
  Conv pu1/1 -> Vabc pu1/1
  Power Factor Block1/5("PFabc ") -> Power Factor1/1
  Power Factor Block1/2(Qabc) -> Measurement1/2
  Power Factor Block1/3(Vabc y Vabc (rms)) -> Conv pu1/1, Measurement1/3

== system Model_14Bus_AC_DC_Microgrid/Load_4 ==
  note: C
  note: B
  note: A
  note: C
  note: Linea - Neutro
  note: B
  note: A
  Conv pu1 : Gain  Gain=sqrt (3) /Vnom_prim  SaturateOnIntegerOverflow=on  OutDataTypeStr=Inherit: Same as input  ParamDataTypeStr=Inherit: Same as input
  Measurement1 : Scope  NumInputPorts=4
      settings: SampleTime=Ts  Title=Active Powers (W)  ActiveDisplayYMinimum=-49681.18717  ActiveDisplayYMaximum=447130.68457  DataLoggingVariableName=ScopeData17  DataLoggingSaveFormat=Array
  Power Factor Block1 : Subsystem  mask(Power Factor Block){Freq=Fnom, Vinit=[0, 0], Iinit=[0, 0], Ts=0}
      mask prompts: Freq "Fundamental frequency (Hz):"; Vinit "Voltage initial input [ Mag, Phase (degrees) ]:"; Iinit "Current initial input [ Mag, Phase (degrees) ]:"; Ts "Sample time:"
      mask help:
      | Power Factor Block developed by Dr Rodney Tan
      | Version 1.01 (Aug 2016)
      |
      | Compute power factor and phase angle of AC circuit voltage-current pair at fundamental frequency.
      |
      | The computation is based on Power block and Complex number function block.
      |
      | For the first cycle of simulation, the outputs are held constant to the powers computed for the Voltage initial input and Current initial input parameters.
      mask Help:
      | <b>Fundamental Frequency (Hz)</b>
      | Specify the measurement fundamental frequency, in hertz, of the input signal.
      | 
      | <b>Voltage initial input [ Mag, Phase (degrees) ]</b>
      | Specify the voltage initial magnitude and phase to set a constant output for the first cycle of simulation.
      | 
      | <b>Current initial input [ Mag, Phase (degrees) ]</b>
      | Specify the current initial magnitude and phase to set a constant output for the first cycle of simulation.
      | 
      | <b>Sample Time</b>
      | Specify the sample time of the block, in seconds. Set to 0 to implement a continuous block.
      mask TypeOptions Freq: Power/Freq
      mask TypeOptions Vinit: Power/Vinit
      mask TypeOptions Iinit: Power/Iinit
      mask TypeOptions Ts: Power/Ts
  Power Factor1 : Display
  THD : spsTHDLib/THD  Freq=60  Ts=Ts_Power
  THD (% and signal) : Scope  NumInputPorts=2
      settings: TimeSpan=0.1  ActiveDisplayYMinimum=-236.74679  ActiveDisplayYMaximum=236.7544  DataLoggingVariableName=ScopeData13
  THD (%) : Display
      settings: Format=bank
  Vabc pu1 : Scope
      settings: TimeSpan=3  Title=Vabc_Instantaneo y rms (pu)  ActiveDisplayYMinimum=-92.95984  ActiveDisplayYMaximum=97.6999  DataLoggingVariableName=ScopeData18
  to % : Gain  Gain=100  SampleTime=Ts_Power
  wires:
  [Iabc_load_14_1] -> Power Factor Block1/2(Iabc)
  [Vabc_load_14_1] -> Power Factor Block1/1(Vabc), THD/1, THD (% and signal)/1  "Signal Vabc"
  THD/1 -> to %/1
  to %/1 -> THD (%)/1, THD (% and signal)/2  "THD (%)"
  Power Factor Block1/4(Iabc y Iabc (rms)) -> Measurement1/4
  Power Factor Block1/1(Pabc) -> Measurement1/1
  Conv pu1/1 -> Vabc pu1/1
  Power Factor Block1/5("PFabc ") -> Power Factor1/1
  Power Factor Block1/2(Qabc) -> Measurement1/2
  Power Factor Block1/3(Vabc y Vabc (rms)) -> Conv pu1/1, Measurement1/3

== system Model_14Bus_AC_DC_Microgrid/Main Grid 69 kV Inf ==
  note: Thevenin equivalent
  69kV 100 MVA 1 : spsThreePhaseSeriesRLCBranchLib/Three-Phase Series RLC Branch  LConnTagsString=A|B|C  RConnTagsString=A|B|C  BranchType=RL  Resistance=69e3^2/100e6/10  Inductance=69e3^2/100e6/(2*pi*60)  Capacitance=1.0  Measurements=None
  Ground1 : spsGroundLib/Ground  LConnTagsString=a
  Programmable Voltage Source1 : spsThreePhaseProgrammableVoltageSourceLib/Three-Phase Programmable Voltage Source  PositiveSequence="[69e3 0  60]"  VariationEntity=None  VariationType=Table of time-amplitude pairs  VariationTypeAlt=Step  VariationStep=-0.3  VariationRate=0.5  VariationMagnitude=0.4  VariationFrequency=2  VariationTiming=[0.1 1.2]  VariationPhaseA=off  Amplitudes=[1]  TimeValues=[0]  HarmonicGeneration=off  HarmonicA=[3 0.2 -25 0]  HarmonicB="[2 0.15  35 2]"  Timing="[0.1  0.6]"  BusType=swing  Pref=500  Qref=0  Qmin=-inf  Qmax=inf
  C : PMIOPort  Side=Right
  B : PMIOPort  Port=2  Side=Right
  A : PMIOPort  Port=3  Side=Right
  connections:
  Programmable Voltage Source1/RConn3 -- 69kV 100 MVA 1/LConn3
  Ground1/LConn1 -- Programmable Voltage Source1/LConn1
  Programmable Voltage Source1/RConn2 -- 69kV 100 MVA 1/LConn2
  69kV 100 MVA 1/LConn1 -- Programmable Voltage Source1/RConn1
  69kV 100 MVA 1/RConn3 -- C/RConn1
  69kV 100 MVA 1/RConn2 -- B/RConn1
  69kV 100 MVA 1/RConn1 -- A/RConn1

== system Model_14Bus_AC_DC_Microgrid/Non Linear AC  Load 9 ==
  Display : Display
  Mean : spsMeanLib/Mean  Freq=10  Vinit=0  Ts=0
  No lineal AC Load 320Kw : spsUniversalBridgeLib/Universal Bridge  Arms=3  SnubberResistance=1e5  SnubberCapacitance=inf  Device=Thyristors  Ron=1e-3  Lon=0  ForwardVoltages="[  0  0  ]"  ForwardVoltage=0  GTOparameters=[ 10e-6 , 20e-6 ]  IGBTparameters=[ 1e-6 , 2e-6 ]  Measurements=None  Measurements_2=None  converterType=Rectifier
  PWM Generator (2-Level) : spsPWMGenerator2LevelLib/PWM Generator (2-Level)  ModulatorType=Three-phase bridge (6 pulses)  ModulatorMode=Unsynchronized  Fc=4080  Pc=0  nF=27  MinMax="[ -1  1 ]"  SamplingTechnique=Natural  ModulatingSignals=on  m=0.8  Freq=Fnom  Phase=-30  Ts=0  ShowCarrierOutport=off
  RL : spsSeriesRLCBranchLib/Series RLC Branch  LConnTagsString=__new0  RConnTagsString=__new0  BranchType=R  Resistance=R_Load_9  Inductance=5e-3  SetiL0=off  InitialCurrent=0  Capacitance=1e-6  Setx0=off  InitialVoltage=0  Measurements=None
  RL1 : spsSeriesRLCBranchLib/Series RLC Branch  LConnTagsString=__new0  RConnTagsString=__new0  BranchType=C  Resistance=1  Inductance=5e-3  SetiL0=off  InitialCurrent=0  Capacitance=10e-6  Setx0=off  InitialVoltage=0  Measurements=None
  "Vdc " : spsVoltageMeasurementLib/Voltage Measurement  Tag=PoWeRsYsTeMmEaSuReMeNt  PhasorSimulation=off  OutputType=Magnitude  PSBequivalent=0
  A : PMIOPort  Tag=PMCPort  Side=Left
  B : PMIOPort  Tag=PMCPort  Port=2  Side=Left
  C : PMIOPort  Tag=PMCPort  Port=3  Side=Left
  wires:
  PWM Generator (2-Level)/1 -> No lineal AC Load 320Kw/1
  "Vdc "/1 -> Mean/1
  Mean/1 -> Display/1
  connections:
  No lineal AC Load 320Kw/RConn1 -- "Vdc "/LConn1 -- RL1/LConn1 -- RL/LConn1
  A/RConn1 -- No lineal AC Load 320Kw/LConn1
  C/RConn1 -- No lineal AC Load 320Kw/LConn3
  B/RConn1 -- No lineal AC Load 320Kw/LConn2
  No lineal AC Load 320Kw/RConn2 -- "Vdc "/LConn2 -- RL1/RConn1 -- RL/RConn1

== system Model_14Bus_AC_DC_Microgrid/OP_max // min ==
  Constant1 : Constant  Value=max_min
  OP_max1 : Constant
  OP_min1 : Constant  Value=0
  Switch2 : Switch  Criteria=u2 > Threshold  SaturateOnIntegerOverflow=off  InputSameDT=off
  on / off : Outport  VectorParamsAs1DForOutWhenUnconnected=off
  wires:
  OP_max1/1 -> Switch2/1
  Constant1/1 -> Switch2/2
  OP_min1/1 -> Switch2/3
  Switch2/1 -> on / off/1

== system Model_14Bus_AC_DC_Microgrid/On//off grid bus DC2 OP_max // min1 ==
  Constant1 : Constant  Value=max_min
  OP_max1 : Constant
  OP_min1 : Constant  Value=0
  Switch2 : Switch  Criteria=u2 > Threshold  SaturateOnIntegerOverflow=off  InputSameDT=off
  on / off : Outport  VectorParamsAs1DForOutWhenUnconnected=off
  wires:
  Switch2/1 -> on / off/1
  OP_min1/1 -> Switch2/3
  Constant1/1 -> Switch2/2
  OP_max1/1 -> Switch2/1

== system Model_14Bus_AC_DC_Microgrid/Resource1 ==
  note: http://calculationsolar.com/blog/?cat=2
  Constant1 : Constant  Value=max_min
  Irradiance (W/m^2) : Display
      settings: Format=bank  Decimation=1000
  Irradiance Temp Demand Max : Subsystem  Tag=STV Subsys  LoadFcn=sigbuilder_block('load');  StartFcn=sigbuilder_block('start');  StopFcn=sigbuilder_block('stop');  ClipboardFcn=sigbuilder_block('clipboard');  mask(Sigbuilder block){tuvar=[0:10]}
      mask help: Sigbuilder GUI
      mask init:
      | if ~strcmp(get_param(bdroot(gcbh),'SimulationStatus'),'stopped') tuvar = sigbuilder_block('maskInit'); end
      settings: CopyFcn=sigbuilder_block('copy');  DeleteFcn=sigbuilder_block('delete');  ModelCloseFcn=sigbuilder_block('modelClose');  PreSaveFcn=sigbuilder_block('preSave');  PauseFcn=sigbuilder_block('pause')  ContinueFcn=sigbuilder_block('continue')  NameChangeFcn=sigbuilder_block('namechange');  OpenFcn=sigbuilder_block('open',[0 30 1024.5 488.25 ]);  CloseFcn=sigbuilder_block('close');
      mask Display: plot(0, 0, 100, 100,[2, 2, 32, 32, 2], [68, 8, 8, 68, 68],[32, 2], [38, 38], [32, 19, 2],[53, 60, 44], [32, 17, 17, 2],[16, 16, 31, 31]);txt = getActiveGroup(gcbh);text(2, 100, txt,'verticalAlignment', 'top');
  Irradiance MIn Demand : Constant  Value=0
  Switch2 : Switch  Criteria=u2 > Threshold  SaturateOnIntegerOverflow=off  InputSameDT=off
  Temperature (deg. C) : Display
      settings: Format=bank  Decimation=1000
  Temp : Outport  VectorParamsAs1DForOutWhenUnconnected=off
  Ir : Outport  Port=2  VectorParamsAs1DForOutWhenUnconnected=off
  wires:
  Irradiance Temp Demand Max/1(Ir) -> Switch2/1, Irradiance (W/m^2)/1
  Irradiance Temp Demand Max/2(Temp) -> Temp/1, Temperature (deg. C)/1
  Irradiance MIn Demand/1 -> Switch2/3
  Constant1/1 -> Switch2/2
  Switch2/1 -> Ir/1  "Radiación (kW/m2)"

== system Model_14Bus_AC_DC_Microgrid/Resources ==
  note: http://calculationsolar.com/blog/?cat=2
  Constant1 : Constant  Value=max_min
  Irradiance (W/m^2) : Display
      settings: Format=bank  Decimation=1000
  Irradiance Temp Demand Max : Subsystem  Tag=STV Subsys  LoadFcn=sigbuilder_block('load');  StartFcn=sigbuilder_block('start');  StopFcn=sigbuilder_block('stop');  ClipboardFcn=sigbuilder_block('clipboard');  mask(Sigbuilder block){tuvar=[0:10]}
      mask help: Sigbuilder GUI
      mask init:
      | if ~strcmp(get_param(bdroot(gcbh),'SimulationStatus'),'stopped') tuvar = sigbuilder_block('maskInit'); end
      settings: CopyFcn=sigbuilder_block('copy');  DeleteFcn=sigbuilder_block('delete');  ModelCloseFcn=sigbuilder_block('modelClose');  PreSaveFcn=sigbuilder_block('preSave');  PauseFcn=sigbuilder_block('pause')  ContinueFcn=sigbuilder_block('continue')  NameChangeFcn=sigbuilder_block('namechange');  OpenFcn=sigbuilder_block('open',[0 30 1024.5 488.25 ]);  CloseFcn=sigbuilder_block('close');
      mask Display: plot(0, 0, 100, 100,[2, 2, 32, 32, 2], [68, 8, 8, 68, 68],[32, 2], [38, 38], [32, 19, 2],[53, 60, 44], [32, 17, 17, 2],[16, 16, 31, 31]);txt = getActiveGroup(gcbh);text(2, 100, txt,'verticalAlignment', 'top');
  Irradiance MIn Demand : Constant  Value=0
  Switch2 : Switch  Criteria=u2 > Threshold  SaturateOnIntegerOverflow=off  InputSameDT=off
  Temperature (deg. C) : Display
      settings: Format=bank  Decimation=1000
  Ir2 : Outport  VectorParamsAs1DForOutWhenUnconnected=off
  temp : Outport  Port=2  VectorParamsAs1DForOutWhenUnconnected=off
  wires:
  Constant1/1 -> Switch2/2
  Irradiance Temp Demand Max/2(Temp) -> temp/1, Temperature (deg. C)/1
  Irradiance MIn Demand/1 -> Switch2/3
  Switch2/1 -> Ir2/1  "Radiación (kW/m2)"
  Irradiance Temp Demand Max/1(Ir) -> Switch2/1, Irradiance (W/m^2)/1

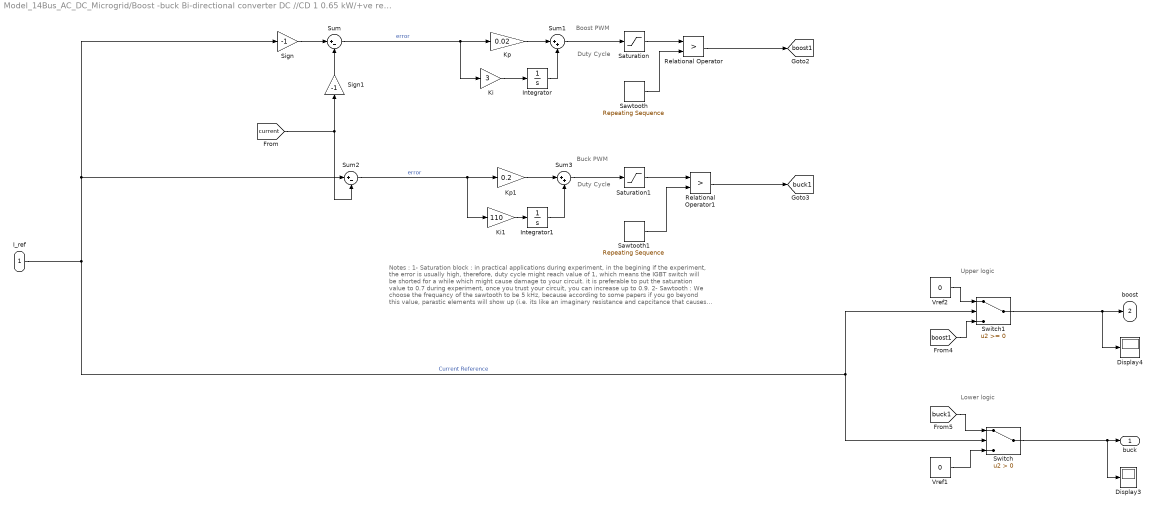
== system Model_14Bus_AC_DC_Microgrid/Boost -buck Bi-directional converter DC //CD 1 0.65 kW/+ve reference For Buck --> -ve reference For Boost <-- ==
  note: Notes :
      | 1- Saturation block : in practical applications during experiment, in the begining if the experiment, the error is usually high, therefore, duty cycle might reach value of 1, which means the IGBT switch will be shorted for a while which might cause damage to your circuit. it is preferable to put the saturation value to 0.7 during experiment, once you trust your circuit, you can increase up to 0.9.
      | 2- Sawtooth : We choose the frequancy of the sawtooth to be 5 kHz, because according to some papers if you go beyond this value, parastic elements will show up (i.e. its like an imaginary resistance and capcitance that causes switching losses and heat). But the more you increase the frequency, the smoother the signal you will get.
      | 3- Step size of your mode l: Make sure that the step size (sample time) in the "model configuration parameters" is smaller than 1/f of the sawtooth. For example, lets say that the sawtooth f = 2 Hz or cycle/sec, meaning the triangle (cycle) repeats every 1/2 sec. Step size or sample time means how many point matlab plot every cycle, lets say it is 1/4 (i.e. plot a point every 0.25 sec), that means that the triangle will be plotted with only two points. That reduce the accuracy, Moreover if the step size is greater than 1/f of the sawtooth, the sawtooth output will be zero.
  note: Buck PWM
  note: Duty Cycle
  note: Upper logic
  note: Lower logic
  note: Boost PWM
  note: Duty Cycle
  I_ref : Inport
  Display3 : Display
  Display4 : Display
  Integrator : Integrator  LimitOutput=on  UpperSaturationLimit=0.9  LowerSaturationLimit=0
  Integrator1 : Integrator  LimitOutput=on  UpperSaturationLimit=0.9  LowerSaturationLimit=0
  Ki : Gain  Gain=3
  Ki1 : Gain  Gain=110
  Kp : Gain  Gain=0.02
  Kp1 : Gain  Gain=0.2
  Relational Operator : RelationalOperator  Operator=>  OutDataTypeStr=boolean  InputSameDT=off
  Relational Operator1 : RelationalOperator  Operator=>  OutDataTypeStr=boolean  InputSameDT=off
  Saturation : Saturate  UpperLimit=0.9  LowerLimit=0
  Saturation1 : Saturate  UpperLimit=0.8  LowerLimit=0
  Sawtooth : simulink/Sources/Repeating Sequence  rep_seq_t=[0 1/5000]  rep_seq_y=[0 1]
  Sawtooth1 : simulink/Sources/Repeating Sequence  rep_seq_t=[0 1/5000]  rep_seq_y=[0 1]
  Sign : Gain  Gain=-1
  Sign1 : Gain  Gain=-1
  Sum : Sum  Inputs=|+-
  Sum1 : Sum  Inputs=|++
  Sum2 : Sum  Inputs=|+-
  Sum3 : Sum  Inputs=|++
  Switch : Switch  Criteria=u2 > Threshold  SaturateOnIntegerOverflow=off  InputSameDT=off
  Switch1 : Switch  SaturateOnIntegerOverflow=off  InputSameDT=off
  Vref1 : Constant  Value=0
  Vref2 : Constant  Value=0
  buck : Outport  VectorParamsAs1DForOutWhenUnconnected=off
  boost : Outport  Port=2  VectorParamsAs1DForOutWhenUnconnected=off
  tag scope: boost1=global, buck1=global
  wires:
  Integrator/1 -> Sum1/2
  Kp/1 -> Sum1/1
  Sum/1 -> Kp/1, Ki/1  "error"
  Relational Operator/1 -> [boost1]
  Sign/1 -> Sum/1
  Sum1/1 -> Saturation/1
  Ki/1 -> Integrator/1
  Sum3/1 -> Saturation1/1
  Integrator1/1 -> Sum3/2
  Sawtooth/1 -> Relational Operator/2
  Sawtooth1/1 -> Relational Operator1/2
  [current] -> Sum2/2, Sign1/1
  Kp1/1 -> Sum3/1
  Relational Operator1/1 -> [buck1]
  Sum2/1 -> Ki1/1, Kp1/1  "error"
  Saturation/1 -> Relational Operator/1
  Saturation1/1 -> Relational Operator1/1
  Ki1/1 -> Integrator1/1
  Vref1/1 -> Switch/3
  Vref2/1 -> Switch1/1
  [boost1] -> Switch1/3
  [buck1] -> Switch/1
  I_ref/1 -> Sum2/1, Sign/1, Switch1/2, Switch/2  "Current Reference"
  Sign1/1 -> Sum/2
  Switch1/1 -> Display4/1, boost/1
  Switch/1 -> Display3/1, buck/1
